simulink model "tank_open_loop"  (R2018b)
settings: Solver=VariableStepAuto  StartTime=0.0  StopTime=10.0  RelTol=1e-3
model workspace (MAT data in the model file):
  A = Simulink.Parameter
  A.Value = 1
  A.DataType = 'auto'
  A.DocUnits = 'm^2'
  A.Dimensions = [1 1]
  h0 = Simulink.Parameter
  h0.Value = 0
  h0.DataType = 'auto'
  h0.DocUnits = '<m>'
  h0.Dimensions = [1 1]
  k1 = Simulink.Parameter
  k1.Value = 10
  k1.DataType = 'auto'
  k1.Dimensions = [1 1]
  qin = Simulink.Parameter
  qin.Value = 0.4
  qin.DataType = 'auto'
  qin.DocUnits = '<m^3/s>'
  qin.Dimensions = [1 1]
settings Model: OrderedModelArguments=off  Creator=waleed.elbadry  LastModifiedBy=waleed.elbadry

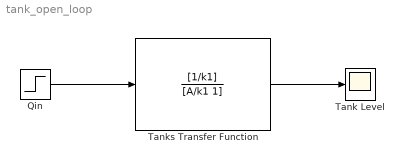
== system tank_open_loop ==
  Qin : Step  Time=0  After=qin  SampleTime=0
  Tank Level : Scope
  Tanks Transfer Function : TransferFcn  Numerator=[1/k1]  Denominator=[A/k1 1]
  wires:
  Qin/1 -> Tanks Transfer Function/1
  Tanks Transfer Function/1 -> Tank Level/1
